simulink model "sim_madrc_completo_v2"  (R2020b)
settings: Solver=VariableStepAuto  StartTime=0.0  StopTime=20000  RelTol=1e-3
values from neighbouring files (symbols this model uses):
  b0 = 0.005    [madrc_2020_completo.m]
  beta1 = 3 * omega_o    (= 2.7)    [madrc_2020_completo.m]
  beta2 = 3 * omega_o^2    (= 2.43)    [madrc_2020_completo.m]
  beta3 = omega_o^3    (= 0.729)    [madrc_2020_completo.m]
  denominador_gcp = conv(den_poly_gcp, conv(den_poly_gcp, den_poly_gcp))    [madrc_2020_completo.m]
  denominador_real = conv(den_poly, conv(den_poly, conv(den_poly, conv(den_poly, den_poly))))    [madrc_2020_completo.m]
  kd = 2 * omega_c    (= 0.044)    [madrc_2020_completo.m]
  kp = omega_c^2    (= 0.000484)    [madrc_2020_completo.m]
  numerador_gcp = 1    [madrc_2020_completo.m]
  numerador_real = K    [madrc_2020_completo.m]
  ref_final = 26,4    [madrc_2020_completo.m]
  ref_inicial = 0    [madrc_2020_completo.m]
  t_degrau = 50    [madrc_2020_completo.m]
  Ts = 1    [madrc_2020_completo.m]
settings Model: Creator=diego  LastModifiedBy=diego

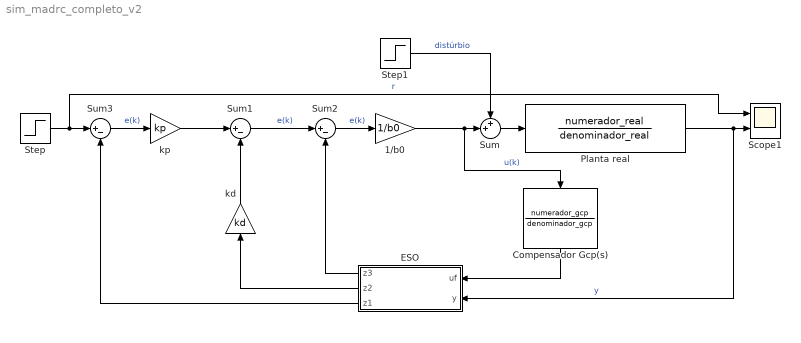
== system sim_madrc_completo_v2 ==
  1/b0 : Gain  Gain=1/b0
  Compensador Gcp(s) : TransferFcn  Numerator=numerador_gcp  Denominator=denominador_gcp
  ESO : Subsystem
  Planta real : TransferFcn  Numerator=numerador_real  Denominator=denominador_real
  Scope1 : Scope  NumInputPorts=2
  Step : Step  Time=t_degrau  Before=ref_inicial  After=ref_final  SampleTime=Ts
  Step1 : Step  Time=10000  After=0.25  SampleTime=Ts
  Sum : Sum  Inputs=++|
  Sum1 : Sum  Inputs=|+-
  Sum2 : Sum  Inputs=|+-
  Sum3 : Sum  Inputs=|+-
  kd : Gain  Gain=kd
  kp : Gain  Gain=kp
  wires:
  Sum3/1 -> kp/1  "e(k)"
  kp/1 -> Sum1/1
  kd/1 -> Sum1/2
  Sum1/1 -> Sum2/1  "e(k)"
  Sum2/1 -> 1/b0/1  "e(k)"
  Step/1 -> Scope1/1, Sum3/1  "r"
  1/b0/1 -> Compensador Gcp(s)/1, Sum/2  "u(k)"
  Step1/1 -> Sum/1  "distúrbio"
  Sum/1 -> Planta real/1
  Planta real/1 -> ESO/2(y), Scope1/2  "y"
  ESO/3(z1) -> Sum3/2
  ESO/2(z2) -> kd/1
  ESO/1(z3) -> Sum2/2
  Compensador Gcp(s)/1 -> ESO/1(uf)

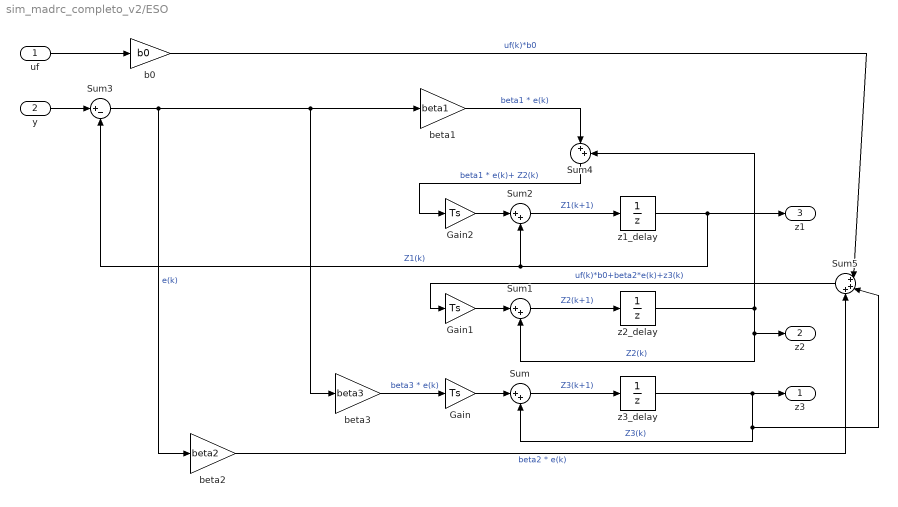
== system sim_madrc_completo_v2/ESO ==
  uf : Inport
  y : Inport  Port=2
  Gain : Gain  Gain=Ts
  Gain1 : Gain  Gain=Ts
  Gain2 : Gain  Gain=Ts
  Sum{,1..2,4} (4 alike) : Sum  Inputs=|++
  Sum3 : Sum  Inputs=|+-
  Sum5 : Sum  Inputs=|+++
  b0 : Gain  Gain=b0
  beta1 : Gain  Gain=beta1
  beta2 : Gain  Gain=beta2
  beta3 : Gain  Gain=beta3
  z1_delay : UnitDelay  SampleTime=-1  HasFrameUpgradeWarning=on
  z2_delay : UnitDelay  SampleTime=-1  HasFrameUpgradeWarning=on
  z3_delay : UnitDelay  SampleTime=-1  HasFrameUpgradeWarning=on
  z3 : Outport
  z2 : Outport  Port=2
  z1 : Outport  Port=3
  wires:
  Sum3/1 -> beta1/1, beta3/1, beta2/1  "e(k)"
  Sum5/1 -> Gain1/1  "uf(k)*b0+beta2*e(k)+z3(k)"
  beta2/1 -> Sum5/3  "beta2 * e(k)"
  z1_delay/1 -> z1/1, Sum3/2, Sum2/2  "Z1(k)"
  Gain1/1 -> Sum1/1
  Gain2/1 -> Sum2/1
  Sum2/1 -> z1_delay/1  "Z1(k+1)"
  beta3/1 -> Gain/1  "beta3 * e(k)"
  Sum4/1 -> Gain2/1  "beta1 * e(k)+ Z2(k)"
  beta1/1 -> Sum4/1  "beta1 * e(k)"
  Gain/1 -> Sum/1
  z3_delay/1 -> Sum5/2, Sum/2, z3/1  "Z3(k)"
  Sum1/1 -> z2_delay/1  "Z2(k+1)"
  z2_delay/1 -> z2/1, Sum1/2, Sum4/2  "Z2(k)"
  Sum/1 -> z3_delay/1  "Z3(k+1)"
  y/1 -> Sum3/1
  uf/1 -> b0/1
  b0/1 -> Sum5/1  "uf(k)*b0"
